simulink subsystem "PID"  (R2026a)
settings: Solver=VariableStepAuto
settings Model: Creator=louis  LastModifiedBy=louis

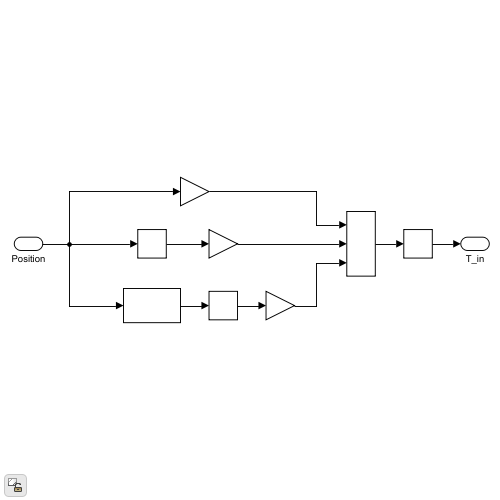
[thumbnail: Simulink's stored preview of the top-level diagram]
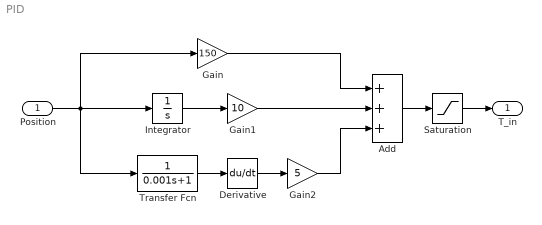
== system PID ==
  Position : Inport
  Add : Sum  Inputs=+++
  Derivative : Derivative
  Gain : Gain  Gain=150
  Gain1 : Gain  Gain=10
  Gain2 : Gain  Gain=5
  Integrator : Integrator
  Saturation : Saturate  UpperLimit=3.82  LowerLimit=-3.82
  Transfer Fcn : TransferFcn  Denominator=[0.001 1]
  T_in : Outport
  wires:
  Position/1 -> Gain/1, Integrator/1, Transfer Fcn/1
  Integrator/1 -> Gain1/1
  Gain1/1 -> Add/2
  Gain/1 -> Add/1
  Transfer Fcn/1 -> Derivative/1
  Gain2/1 -> Add/3
  Derivative/1 -> Gain2/1
  Saturation/1 -> T_in/1
  Add/1 -> Saturation/1
